simulink model "no_connections_stacey"  (R2023b)
settings: Solver=VariableStepAuto  StartTime=0.0  StopTime=20  RelTol=1e-3
undefined symbols (not defined in the file): delta_f, FF_gain, Fx200lbf, g, Izz, Kd, Ki, Kp, L, Lf, Lr, r_d_term, s, s_desired, T_down, T_request, T_switch, T_up, Tm_max, TV_switch, TV_vel_trig
libraries: slpidlib x2, Solver_SF x1, simulink x1, fuzblock x1
settings Model: Creator=savchenko.6  LastModifiedBy=savchenko.6
settings DataIOCC: ReturnWorkspaceOutputs=off
settings OptimizationCC: ReuseModelBlockBuffer=off

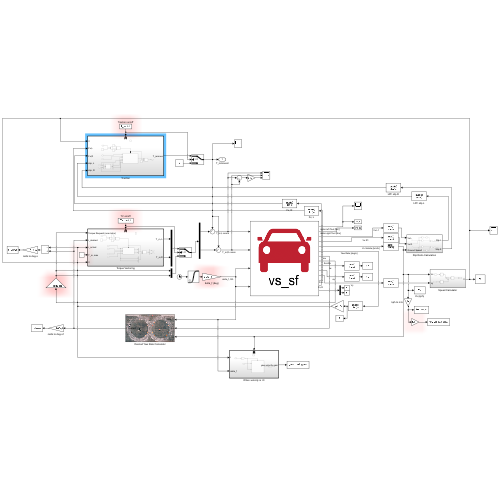
[thumbnail: Simulink's stored preview of the top-level diagram]
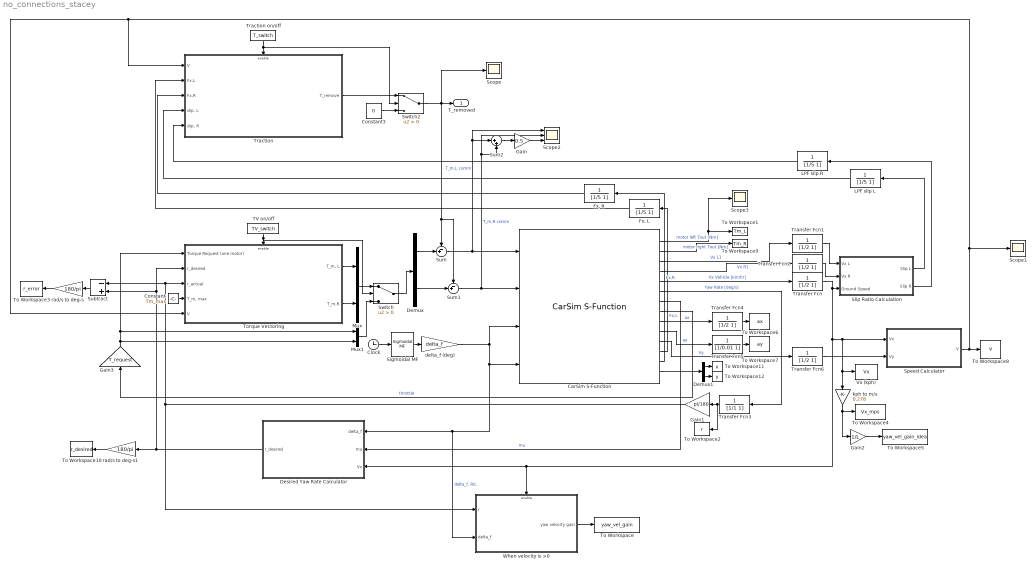
== system no_connections_stacey ==
  CarSim S-Function : Solver_SF/CarSim S-Function  Priority=1  SIMFILE=simfile.sim  Run_RTs=off  vs_state_ind=Run  StopMode_ind=Vehicle Model
  Clock : Clock
  Constant : Constant  Value=Tm_max
  Constant3 : Constant  Value=0
  Demux : Demux  Outputs=2
  Demux1 : Demux  Outputs=2
  Desired Yaw Rate Calculator : Subsystem
      mask Display: image('\\coeit.osu.edu\home\s\savchenko.6\Desktop\Capstone\Post-Depression\FB2018_Skidpad.png'); % Use "Edit Image" on toolstrip to change.
  "Fx, L" : TransferFcn  Denominator=[1/5 1]
  "Fx, R" : TransferFcn  Denominator=[1/5 1]
  Gain : Gain  Gain=0.5
  Gain1 : Gain  Gain=pi/180
  Gain2 : Gain  Gain=1/L
  Gain3 : Gain  Gain=T_request
  LPF slip L : TransferFcn  Denominator=[1/5 1]
  LPF slip R : TransferFcn  Denominator=[1/5 1]
  Mux : Mux  Inputs=2
  Mux1 : Mux  Inputs=2
  Scope : Scope
  Scope1 : Scope
  Scope2 : Scope  NumInputPorts=3
  Scope3 : Scope
  Sigmoidal MF : fuzblock/Membership  Functions/Sigmoidal MF  a=10  c=0.5
  Slip Ratio Calculation : Subsystem
  Speed Calculator : Subsystem
  Subtract : Sum  Inputs=-+
  Sum : Sum  Inputs=-+|
  Sum1 : Sum  Inputs=-+|
  Sum2 : Sum  Inputs=|++
  Switch : Switch  Criteria=u2 > Threshold  SaturateOnIntegerOverflow=off  InputSameDT=off
  Switch2 : Switch  Criteria=u2 > Threshold  SaturateOnIntegerOverflow=off  InputSameDT=off
  TV on/off : Constant  Value=TV_switch
  To Workspace : ToWorkspace  VariableName=yaw_vel_gain  SampleTime=-1
  To Workspace1 : ToWorkspace  VariableName=Tm_L  SampleTime=-1
  To Workspace10 : ToWorkspace  VariableName=r_desired  SampleTime=-1
  To Workspace11 : ToWorkspace  VariableName=x  SampleTime=-1
  To Workspace12 : ToWorkspace  VariableName=y  SampleTime=-1
  To Workspace2 : ToWorkspace  VariableName=r  SampleTime=-1
  To Workspace3 : ToWorkspace  VariableName=r_error  SampleTime=-1
  To Workspace4 : ToWorkspace  VariableName=Vx_mps  SampleTime=-1
  To Workspace5 : ToWorkspace  VariableName=yaw_vel_gain_ideal  SampleTime=-1
  To Workspace6 : ToWorkspace  VariableName=ax  SampleTime=-1
  To Workspace7 : ToWorkspace  VariableName=ay  SampleTime=-1
  To Workspace8 : ToWorkspace  VariableName=V  SampleTime=-1
  To Workspace9 : ToWorkspace  VariableName=Tm_R  SampleTime=-1
  Torque Vectoring : Subsystem  TreatAsAtomicUnit=on
  Traction : Subsystem  TreatAsAtomicUnit=on
  Traction on/off : Constant  Value=T_switch
  Transfer Fcn{,1..2,4,6} (5 alike) : TransferFcn  Denominator=[1/2 1]
  Transfer Fcn3 : TransferFcn  Denominator=[1/1 1]
  Transfer Fcn5 : TransferFcn  Denominator=[1/0.01 1]
  Vx (kph) : ToWorkspace  VariableName=Vx  SampleTime=-1
  When velocity is >0 : Subsystem  TreatAsAtomicUnit=on
  delta_f (deg) : Gain  Gain=delta_f
  kph to m/s : Gain  Gain=0.278
  rad/s to deg-s : Gain  Gain=180/pi
  rad/s to deg-s1 : Gain  Gain=180/pi
  T_removed : Outport
  wires:
  CarSim S-Function/5 -> Transfer Fcn/1  "Vx Vehicle [km/hr]"
  CarSim S-Function/6 -> Transfer Fcn3/1  "Yaw Rate [deg/s]"
  CarSim S-Function/7 -> Desired Yaw Rate Calculator/2(mu)  "mu"
  CarSim S-Function/3 -> Transfer Fcn1/1  "Vx L1"
  CarSim S-Function/4 -> Transfer Fcn2/1  "Vx R1"
  Slip Ratio Calculation/1(Slip L) -> LPF slip L/1
  Transfer Fcn/1 -> Speed Calculator/1(Vx), kph to m/s/1, Vx (kph)/1, Desired Yaw Rate Calculator/3(Vx), When velocity is >0/Enable, Slip Ratio Calculation/3(Ground Speed)
  Transfer Fcn1/1 -> Slip Ratio Calculation/1(Vx L)
  Transfer Fcn2/1 -> Slip Ratio Calculation/2(Vx R)
  TV on/off/1 -> Switch/2, Torque Vectoring/Enable
  Constant/1 -> Torque Vectoring/4("T_m, max")
  Torque Vectoring/2(T_m,R) -> Mux/2
  Torque Vectoring/1("T_m, L") -> Mux/1
  Mux/1 -> Switch/1
  Switch/1 -> Demux/1
  Mux1/1 -> Switch/3
  CarSim S-Function/8 -> Gain3/1  "throttle"
  When velocity is >0/1(yaw velocity gain) -> To Workspace/1
  Gain2/1 -> To Workspace5/1
  kph to m/s/1 -> Gain2/1, To Workspace4/1
  Subtract/1 -> rad/s to deg-s/1
  Gain3/1 -> Mux1/2, Mux1/1, Torque Vectoring/1(Torque Request (one motor))
  Traction/1(T_remove) -> Switch2/1
  Constant3/1 -> Switch2/3
  Traction on/off/1 -> Switch2/2, Traction/Enable
  Demux/2 -> Sum1/2
  Demux/1 -> Sum/2
  Switch2/1 -> Scope/1, Sum/1, Sum1/1, T_removed/1
  Sum1/1 -> Sum2/2, Scope2/2, CarSim S-Function/2  "T_m,R comm"
  Sum/1 -> Sum2/1, Scope2/1, CarSim S-Function/1  "T_m,L comm"
  CarSim S-Function/9 -> Transfer Fcn4/1  "ax"
  CarSim S-Function/10 -> Transfer Fcn5/1  "ay"
  Slip Ratio Calculation/2(Slip R) -> LPF slip R/1
  LPF slip L/1 -> Traction/4("slip, L")
  LPF slip R/1 -> Traction/5("slip, R")
  Gain1/1 -> When velocity is >0/1(r), Torque Vectoring/3(r_actual), Subtract/1
  Desired Yaw Rate Calculator/1(r_desired) -> rad/s to deg-s1/1, Torque Vectoring/2(r_desired), Subtract/2
  rad/s to deg-s/1 -> To Workspace3/1
  CarSim S-Function/11 -> Transfer Fcn6/1  "Vy"
  Transfer Fcn6/1 -> Speed Calculator/2(Vy)
  Speed Calculator/1(V) -> To Workspace8/1, Scope1/1, Torque Vectoring/5(V), Traction/1(V)
  CarSim S-Function/12 -> "Fx, L"/1  "Fx,L"
  CarSim S-Function/13 -> "Fx, R"/1  "Fx,R"
  Transfer Fcn4/1 -> To Workspace6/1
  Transfer Fcn5/1 -> To Workspace7/1
  CarSim S-Function/2 -> To Workspace9/1  "motor right Tout [Nm]"
  CarSim S-Function/1 -> Scope3/1, To Workspace1/1  "motor left Tout [Nm]"
  "Fx, R"/1 -> Traction/3(Fx,R)
  "Fx, L"/1 -> Traction/2(Fx,L)
  Transfer Fcn3/1 -> To Workspace2/1, Gain1/1
  rad/s to deg-s1/1 -> To Workspace10/1
  CarSim S-Function/14 -> Demux1/1
  Demux1/1 -> To Workspace11/1
  Demux1/2 -> To Workspace12/1
  delta_f (deg)/1 -> CarSim S-Function/3, When velocity is >0/2(delta_f), Desired Yaw Rate Calculator/1("delta_f "), CarSim S-Function/4  "delta_f, R/L"
  Sigmoidal MF/1 -> delta_f (deg)/1
  Clock/1 -> Sigmoidal MF/1
  Sum2/1 -> Gain/1
  Gain/1 -> Scope2/3

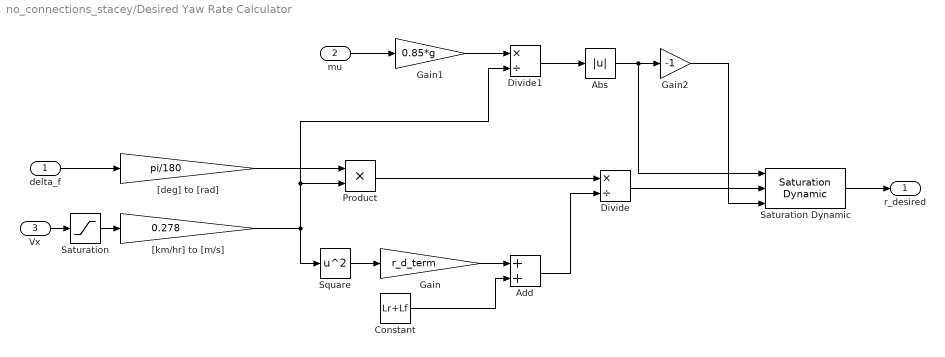
== system no_connections_stacey/Desired Yaw Rate Calculator ==
  "delta_f " : Inport
  mu : Inport  Port=2
  Vx : Inport  Port=3
  Abs : Abs  SaturateOnIntegerOverflow=off
  Add : Sum
  Constant : Constant  Value=Lr+Lf
  Divide : Product  Inputs=*/
  Divide1 : Product  Inputs=*/
  Gain : Gain  Gain=r_d_term
  Gain1 : Gain  Gain=0.85*g
  Gain2 : Gain  Gain=-1
  Product : Product
  Saturation : Saturate  UpperLimit=10000  LowerLimit=0.01
  Saturation Dynamic : simulink/Discontinuities/Saturation Dynamic  OutMin=[]  OutMax=[]  OutDataTypeStr=Inherit: Same as second input  OutDataType=fixdt(1, 16)  OutScaling=2^-10  DoSatur=off
  Square : Math  Operator=square
  "[deg] to [rad]" : Gain  Gain=pi/180
  "[km/hr] to [m/s]" : Gain  Gain=0.278
  r_desired : Outport
  wires:
  "delta_f "/1 -> "[deg] to [rad]"/1
  Vx/1 -> Saturation/1
  Saturation/1 -> "[km/hr] to [m/s]"/1
  "[deg] to [rad]"/1 -> Product/1
  "[km/hr] to [m/s]"/1 -> Square/1, Divide1/2, Product/2
  Product/1 -> Divide/1
  Square/1 -> Gain/1
  Gain/1 -> Add/1
  Constant/1 -> Add/2
  Add/1 -> Divide/2
  Divide/1 -> Saturation Dynamic/2
  Saturation Dynamic/1 -> r_desired/1
  mu/1 -> Gain1/1
  Gain1/1 -> Divide1/1
  Divide1/1 -> Abs/1
  Abs/1 -> Saturation Dynamic/1, Gain2/1
  Gain2/1 -> Saturation Dynamic/3

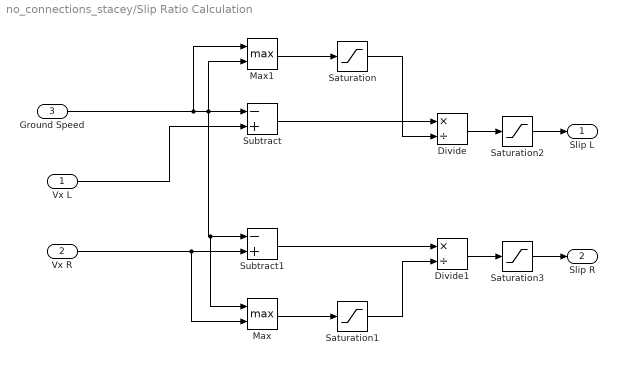
== system no_connections_stacey/Slip Ratio Calculation ==
  Vx L : Inport
  Vx R : Inport  Port=2
  Ground Speed : Inport  Port=3
  Divide : Product  Inputs=*/
  Divide1 : Product  Inputs=*/
  Max : MinMax  Function=max  Inputs=2
  Max1 : MinMax  Function=max  Inputs=2
  Saturation : Saturate  UpperLimit=1000  LowerLimit=0.0001
  Saturation1 : Saturate  UpperLimit=1000  LowerLimit=0.0001
  Saturation2 : Saturate  UpperLimit=1  LowerLimit=0
  Saturation3 : Saturate  UpperLimit=1  LowerLimit=0
  Subtract : Sum  Inputs=-+
  Subtract1 : Sum  Inputs=-+
  Slip L : Outport
  Slip R : Outport  Port=2
  wires:
  Vx L/1 -> Subtract/2
  Vx R/1 -> Max/2, Subtract1/2
  Max1/1 -> Saturation/1
  Max/1 -> Saturation1/1
  Subtract/1 -> Divide/1
  Saturation/1 -> Divide/2
  Subtract1/1 -> Divide1/1
  Saturation1/1 -> Divide1/2
  Divide/1 -> Saturation2/1
  Divide1/1 -> Saturation3/1
  Saturation2/1 -> Slip L/1
  Saturation3/1 -> Slip R/1
  Ground Speed/1 -> Max1/1, Max/1, Subtract1/1, Max1/2, Subtract/1

== system no_connections_stacey/Speed Calculator ==
  Vx : Inport
  Vy : Inport  Port=2
  Sqrt : Sqrt
  Square : Math  Operator=square
  Square1 : Math  Operator=square
  Sum : Sum  Inputs=|++
  V : Outport
  wires:
  Vx/1 -> Square/1
  Vy/1 -> Square1/1
  Square/1 -> Sum/1
  Square1/1 -> Sum/2
  Sum/1 -> Sqrt/1
  Sqrt/1 -> V/1

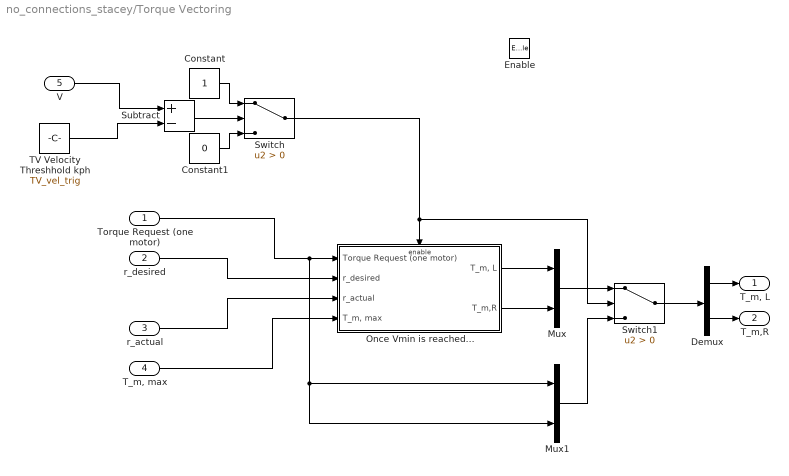
== system no_connections_stacey/Torque Vectoring ==
  Torque Request (one motor) : Inport
  r_desired : Inport  Port=2
  r_actual : Inport  Port=3
  "T_m, max" : Inport  Port=4
  V : Inport  Port=5
  Enable : EnablePort  StatesWhenEnabling=reset
  Constant : Constant
  Constant1 : Constant  Value=0
  Demux : Demux  Outputs=2
  Mux : Mux  Inputs=2
  Mux1 : Mux  Inputs=2
  Once Vmin is reached... : Subsystem
  Subtract : Sum  Inputs=+-
  Switch : Switch  Criteria=u2 > Threshold  SaturateOnIntegerOverflow=off  InputSameDT=off
  Switch1 : Switch  Criteria=u2 > Threshold  SaturateOnIntegerOverflow=off  InputSameDT=off
  TV Velocity Threshhold kph : Constant  Value=TV_vel_trig
  "T_m, L" : Outport
  T_m,R : Outport  Port=2
  wires:
  Torque Request (one motor)/1 -> Mux1/2, Mux1/1, Once Vmin is reached.../1(Torque Request (one motor))
  r_desired/1 -> Once Vmin is reached.../2(r_desired)
  r_actual/1 -> Once Vmin is reached.../3(r_actual)
  "T_m, max"/1 -> Once Vmin is reached.../4("T_m, max")
  Once Vmin is reached.../1("T_m, L") -> Mux/1
  Once Vmin is reached.../2(T_m,R) -> Mux/2
  Mux/1 -> Switch1/1
  Mux1/1 -> Switch1/3
  Switch1/1 -> Demux/1
  Demux/1 -> "T_m, L"/1
  Demux/2 -> T_m,R/1
  Constant1/1 -> Switch/3
  Switch/1 -> Switch1/2, Once Vmin is reached.../Enable
  Constant/1 -> Switch/1
  TV Velocity Threshhold kph/1 -> Subtract/2
  Subtract/1 -> Switch/2
  V/1 -> Subtract/1

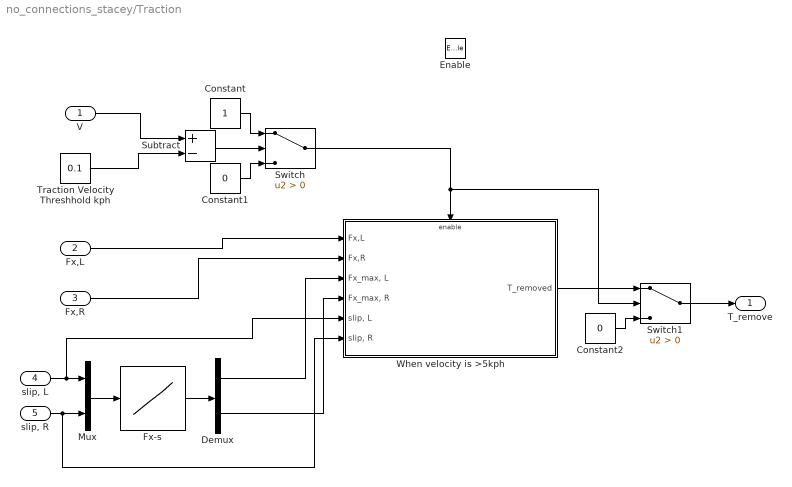
== system no_connections_stacey/Traction ==
  V : Inport
  Fx,L : Inport  Port=2
  Fx,R : Inport  Port=3
  "slip, L" : Inport  Port=4
  "slip, R" : Inport  Port=5
  Enable : EnablePort  StatesWhenEnabling=reset
  Constant : Constant
  Constant1 : Constant  Value=0
  Constant2 : Constant  Value=0
  Demux : Demux  Outputs=2
  Fx-s : Lookup_n-D  NumberOfTableDimensions=1  BreakpointsForDimension1=s  Table=Fx200lbf  InternalRulePriority=Speed  RndMeth=Simplest
  Mux : Mux  Inputs=2
  Subtract : Sum  Inputs=+-
  Switch : Switch  Criteria=u2 > Threshold  SaturateOnIntegerOverflow=off  InputSameDT=off
  Switch1 : Switch  Criteria=u2 > Threshold  SaturateOnIntegerOverflow=off  InputSameDT=off
  Traction Velocity Threshhold kph : Constant  Value=0.1
  When velocity is >5kph : Subsystem  TreatAsAtomicUnit=on
  T_remove : Outport
  wires:
  V/1 -> Subtract/1
  Traction Velocity Threshhold kph/1 -> Subtract/2
  Subtract/1 -> Switch/2
  Constant/1 -> Switch/1
  Constant1/1 -> Switch/3
  Switch/1 -> Switch1/2, When velocity is >5kph/Enable
  "slip, L"/1 -> When velocity is >5kph/5("slip, L"), Mux/1
  "slip, R"/1 -> When velocity is >5kph/6("slip, R"), Mux/2
  Mux/1 -> Fx-s/1
  Fx-s/1 -> Demux/1
  When velocity is >5kph/1(T_removed) -> Switch1/1
  Switch1/1 -> T_remove/1
  Constant2/1 -> Switch1/3
  Fx,L/1 -> When velocity is >5kph/1(Fx,L)
  Fx,R/1 -> When velocity is >5kph/2(Fx,R)
  Demux/1 -> When velocity is >5kph/3("Fx_max, L")
  Demux/2 -> When velocity is >5kph/4("Fx_max, R")

== system no_connections_stacey/When velocity is >0 ==
  r : Inport
  delta_f : Inport  Port=2
  Enable : EnablePort  StatesWhenEnabling=reset
  When Steering : Subsystem  TreatAsAtomicUnit=on
  deg to rad : Gain  Gain=pi/180
  yaw velocity gain : Outport
  wires:
  delta_f/1 -> deg to rad/1
  r/1 -> When Steering/1(r)
  When Steering/1(yaw velocity gain) -> yaw velocity gain/1
  deg to rad/1 -> When Steering/2(delta_f), When Steering/Enable

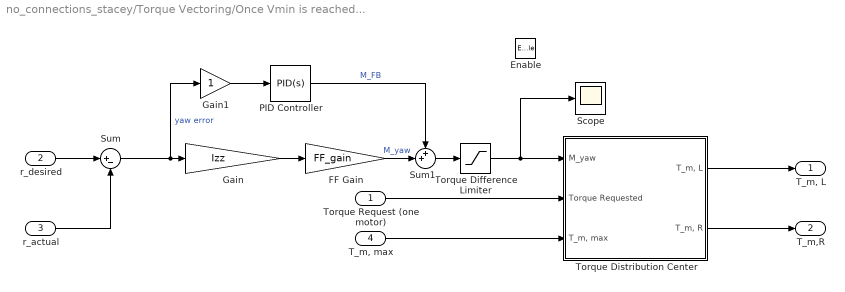
== system no_connections_stacey/Torque Vectoring/Once Vmin is reached... ==
  Torque Request (one motor) : Inport
  r_desired : Inport  Port=2
  r_actual : Inport  Port=3
  "T_m, max" : Inport  Port=4
  Enable : EnablePort  StatesWhenEnabling=reset
  FF Gain : Gain  Gain=FF_gain
  Gain : Gain  Gain=Izz
  Gain1 : Gain
  PID Controller : slpidlib/PID Controller  Controller=PID  Form=Parallel  TimeDomain=Continuous-time  UseExternalTs=off  SampleTime=-1  IntegratorMethod=Forward Euler  FilterMethod=Forward Euler  ControllerParametersSource=internal  P=Kp  I=Ki  UseKiTs=off  D=Kd  N=100  UseFilter=on  TunerSelectOption=Transfer Function Based (PID Tuner App)  InitialConditionSource=internal  InitialConditionForIntegrator=0  InitialConditionForFilter=0  DifferentiatorICPrevScaledInput=0  ExternalReset=none  TrackingMode=off  Kt=1  LimitOutput=off  SatLimitsSource=internal  UpperSaturationLimit=inf  LowerSaturationLimit=-inf  LinearizeAsGain=on  AntiWindupMode=none  Kb=1  LimitIntegrator=off  UpperIntegratorSaturationLimit=inf  LowerIntegratorSaturationLimit=-inf  POutMin=[]  POutMax=[]  IOutMin=[]  IOutMax=[]  DOutMin=[]  DOutMax=[]  NOutMin=[]  NOutMax=[]  SumOutMin=[]  SumOutMax=[]  SaturationOutMin=[]  SaturationOutMax=[]  PParamMin=[]  PParamMax=[]  IParamMin=[]  IParamMax=[]  DParamMin=[]  DParamMax=[]  NParamMin=[]  NParamMax=[]  KbParamMin=[]  KbParamMax=[]  KtParamMin=[]  KtParamMax=[]  KbOutMin=[]  KbOutMax=[]  KtOutMin=[]  KtOutMax=[]  IntegratorOutMin=[]  IntegratorOutMax=[]  FilterOutMin=[]  FilterOutMax=[]  SumI1OutMin=[]  SumI1OutMax=[]  SumI2OutMin=[]  SumI2OutMax=[]  SumI3OutMin=[]  SumI3OutMax=[]  SumI4OutMin=[]  SumI4OutMax=[]  SumDOutMin=[]  SumDOutMax=[]  DifferentiatorOutMin=[]  DifferentiatorOutMax=[]  FilterDiffOutCoefMin=[]  FilterDiffOutCoefMax=[]  ReciprocalOutMin=[]  ReciprocalOutMax=[]  SumDenOutMin=[]  SumDenOutMax=[]  SumNumOutMin=[]  SumNumOutMax=[]  DivideOutMin=[]  DivideOutMax=[]  UdiffTsProdOutMin=[]  UdiffTsProdOutMax=[]  NTsProdOutMin=[]  NTsProdOutMax=[]  UintegralTsProdOutMin=[]  UintegralTsProdOutMax=[]  UngainTsProdOutMin=[]  UngainTsProdOutMax=[]  ClampingZeroOutDataTypeStr=Inherit: Inherit via back propagation  ClampingZeroOutMin=[]  ClampingZeroOutMax=[]  FilterDenConstantOutDataTypeStr=Inherit: Inherit via back propagation  FilterDenConstantOutMin=[]  FilterDenConstantOutMax=[]  PCopyOutDataTypeStr=Inherit: Inherit via back propagation  PCopyOutMin=[]  PCopyOutMax=[]  NCopyOutDataTypeStr=Inherit: Inherit via back propagation  NCopyOutMin=[]  NCopyOutMax=[]  IntegratorContinuousStateAttributes=''  IntegratorStateMustResolveToSignalObject=off  IntegratorRTWStateStorageClass=Auto  FilterContinuousStateAttributes=''  FilterStateMustResolveToSignalObject=off  FilterRTWStateStorageClass=Auto  ParallelPVariant=InternalParameters  IdealPVariant=Disabled  IVariant=InternalParameters  DVariant=InternalParameters  IntegratorVariant=Continuous  SatVariant=Disabled  AWVariant=Passthrough  PCopyVariant=Disabled  TRVariant=Disabled  FdbkBlocksVariant=Forward  IdealPFdbkVariant=Disabled  SatFdbkVariant=Disabled  DerivativeFilterVariant=ContFilter  NVariant=InternalParameters  NCopyVariant=Disabled  FilterICVariant=InternalICsFilter  IntegratorICVariant=InternalICs  ExternalResetVariant=Disabled  TRSumVariant=Passthrough  SumFdbkVariant=Disabled  SumVariant=Sum_PID  TsampFilterVariant=InternalTs  TsampNgainVariant=Passthrough  TsampIntegralVariant=Disabled_SignalSpec  ExternalSaturationOutDataTypeStr=Inherit: Same as second input
  Scope : Scope
  Sum : Sum  Inputs=|+-
  Sum1 : Sum  Inputs=++|
  Torque Difference Limiter : Saturate  UpperLimit=T_up  LowerLimit=T_down
  Torque Distribution Center : Subsystem
  "T_m, L" : Outport
  T_m,R : Outport  Port=2
  wires:
  Torque Request (one motor)/1 -> Torque Distribution Center/2(Torque Requested)
  Gain/1 -> FF Gain/1
  Torque Difference Limiter/1 -> Scope/1, Torque Distribution Center/1(M_yaw)
  r_desired/1 -> Sum/1
  Torque Distribution Center/2("T_m, R") -> T_m,R/1
  Sum/1 -> Gain/1, Gain1/1  "yaw error"
  "T_m, max"/1 -> Torque Distribution Center/3("T_m, max")
  r_actual/1 -> Sum/2
  Torque Distribution Center/1("T_m, L") -> "T_m, L"/1
  Sum1/1 -> Torque Difference Limiter/1
  FF Gain/1 -> Sum1/2  "M_yaw"
  PID Controller/1 -> Sum1/1  "M_FB"
  Gain1/1 -> PID Controller/1

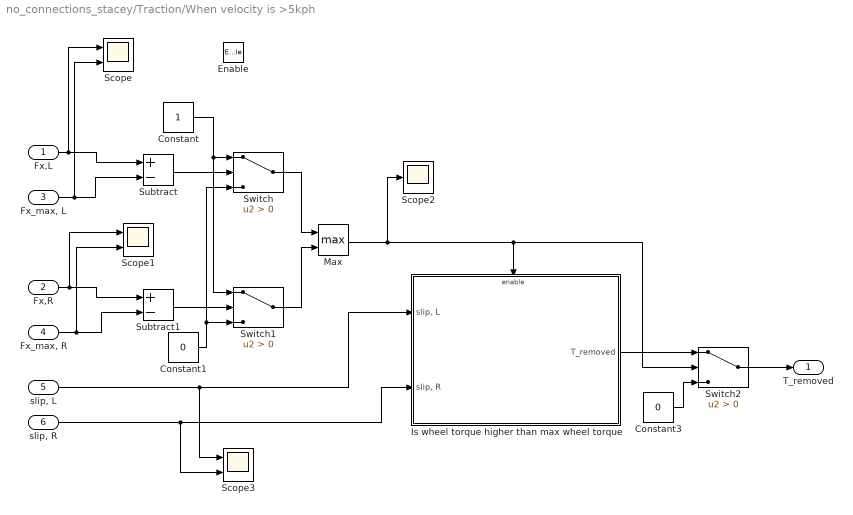
== system no_connections_stacey/Traction/When velocity is >5kph ==
  Fx,L : Inport
  Fx,R : Inport  Port=2
  "Fx_max, L" : Inport  Port=3
  "Fx_max, R" : Inport  Port=4
  "slip, L" : Inport  Port=5
  "slip, R" : Inport  Port=6
  Enable : EnablePort  StatesWhenEnabling=reset
  Constant : Constant
  Constant1 : Constant  Value=0
  Constant3 : Constant  Value=0
  Is wheel torque higher than max wheel torque : Subsystem  TreatAsAtomicUnit=on
  Max : MinMax  Function=max  Inputs=2
  Scope : Scope  NumInputPorts=2
  Scope1 : Scope  NumInputPorts=2
  Scope2 : Scope
  Scope3 : Scope  NumInputPorts=2
  Subtract : Sum  Inputs=+-
  Subtract1 : Sum  Inputs=+-
  Switch : Switch  Criteria=u2 > Threshold  SaturateOnIntegerOverflow=off  InputSameDT=off
  Switch1 : Switch  Criteria=u2 > Threshold  SaturateOnIntegerOverflow=off  InputSameDT=off
  Switch2 : Switch  Criteria=u2 > Threshold  SaturateOnIntegerOverflow=off  InputSameDT=off
  T_removed : Outport
  wires:
  Fx,L/1 -> Scope/1, Subtract/1
  "Fx_max, L"/1 -> Scope/2, Subtract/2
  "Fx_max, R"/1 -> Scope1/2, Subtract1/2
  Fx,R/1 -> Scope1/1, Subtract1/1
  Subtract/1 -> Switch/2
  Subtract1/1 -> Switch1/2
  Constant/1 -> Switch/1, Switch1/1
  Constant1/1 -> Switch1/3, Switch/3
  Switch/1 -> Max/1
  Switch1/1 -> Max/2
  Is wheel torque higher than max wheel torque/1(T_removed) -> Switch2/1
  Constant3/1 -> Switch2/3
  Max/1 -> Scope2/1, Is wheel torque higher than max wheel torque/Enable, Switch2/2
  Switch2/1 -> T_removed/1
  "slip, R"/1 -> Scope3/2, Is wheel torque higher than max wheel torque/2("slip, R")
  "slip, L"/1 -> Is wheel torque higher than max wheel torque/1("slip, L"), Scope3/1

== system no_connections_stacey/When velocity is >0/When Steering ==
  r : Inport
  delta_f : Inport  Port=2
  Enable : EnablePort  StatesWhenEnabling=reset
  Divide : Product  Inputs=*/
  yaw velocity gain : Outport
  wires:
  r/1 -> Divide/1
  delta_f/1 -> Divide/2
  Divide/1 -> yaw velocity gain/1

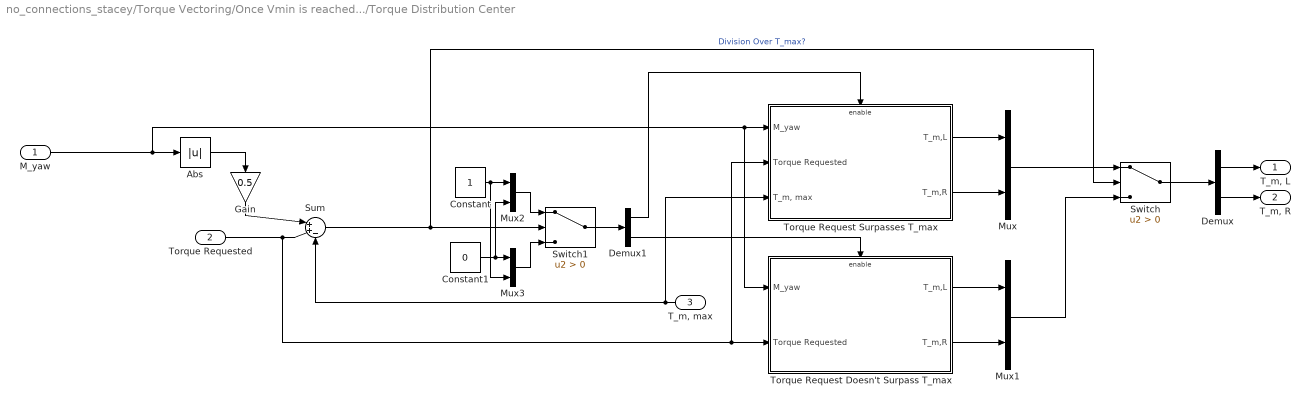
== system no_connections_stacey/Torque Vectoring/Once Vmin is reached.../Torque Distribution Center ==
  M_yaw : Inport
  Torque Requested : Inport  Port=2
  "T_m, max" : Inport  Port=3
  Abs : Abs  SaturateOnIntegerOverflow=off
  Constant : Constant
  Constant1 : Constant  Value=0
  Demux : Demux  Outputs=2
  Demux1 : Demux  Outputs=2
  Gain : Gain  Gain=0.5
  Mux{,1..3} (4 alike) : Mux  Inputs=2
  Sum : Sum  Inputs=|++-
  Switch : Switch  Criteria=u2 > Threshold  SaturateOnIntegerOverflow=off  InputSameDT=off
  Switch1 : Switch  Criteria=u2 > Threshold  SaturateOnIntegerOverflow=off  InputSameDT=off
  Torque Request Doesn't Surpass T_max : Subsystem  TreatAsAtomicUnit=on
  Torque Request Surpasses T_max : Subsystem  TreatAsAtomicUnit=on
  "T_m, L" : Outport
  "T_m, R" : Outport  Port=2
  wires:
  Sum/1 -> Switch1/2, Switch/2  "Division Over T_max?"
  Gain/1 -> Sum/1
  Abs/1 -> Gain/1
  Torque Request Surpasses T_max/1(T_m,L) -> Mux/1
  Torque Request Surpasses T_max/2(T_m,R) -> Mux/2
  Torque Request Doesn't Surpass T_max/1(T_m,L) -> Mux1/1
  Torque Request Doesn't Surpass T_max/2(T_m,R) -> Mux1/2
  Mux/1 -> Switch/1
  Mux1/1 -> Switch/3
  Switch/1 -> Demux/1
  Demux/1 -> "T_m, L"/1
  Demux/2 -> "T_m, R"/1
  Torque Requested/1 -> Torque Request Surpasses T_max/2(Torque Requested), Torque Request Doesn't Surpass T_max/2(Torque Requested), Sum/2
  "T_m, max"/1 -> Sum/3, Torque Request Surpasses T_max/3("T_m, max")
  Mux2/1 -> Switch1/1
  Mux3/1 -> Switch1/3
  Switch1/1 -> Demux1/1
  Demux1/1 -> Torque Request Surpasses T_max/Enable
  Demux1/2 -> Torque Request Doesn't Surpass T_max/Enable
  Constant/1 -> Mux2/1, Mux3/2
  Constant1/1 -> Mux2/2, Mux3/1
  M_yaw/1 -> Torque Request Doesn't Surpass T_max/1(M_yaw), Torque Request Surpasses T_max/1(M_yaw), Abs/1

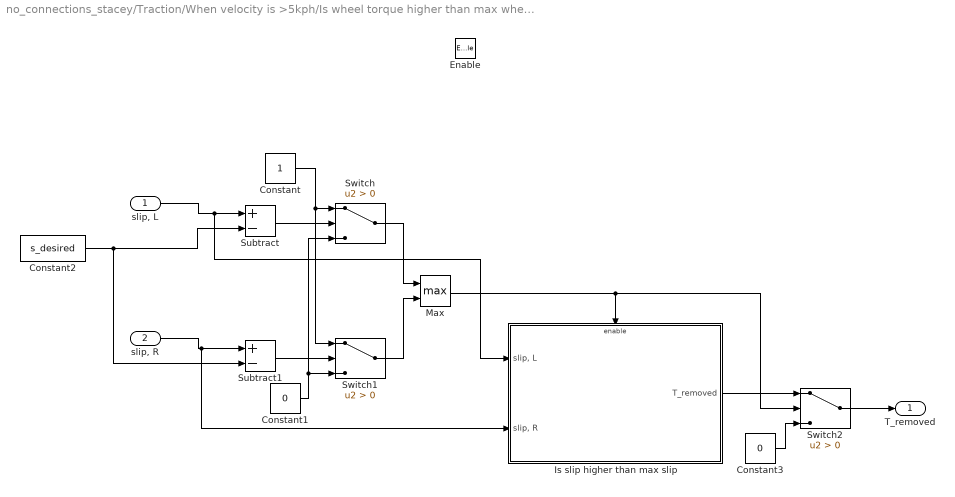
== system no_connections_stacey/Traction/When velocity is >5kph/Is wheel torque higher than max wheel torque ==
  "slip, L" : Inport
  "slip, R" : Inport  Port=2
  Enable : EnablePort  StatesWhenEnabling=reset
  Constant : Constant
  Constant1 : Constant  Value=0
  Constant2 : Constant  Value=s_desired
  Constant3 : Constant  Value=0
  Is slip higher than max slip : Subsystem  TreatAsAtomicUnit=on
  Max : MinMax  Function=max  Inputs=2
  Subtract : Sum  Inputs=+-
  Subtract1 : Sum  Inputs=+-
  Switch : Switch  Criteria=u2 > Threshold  SaturateOnIntegerOverflow=off  InputSameDT=off
  Switch1 : Switch  Criteria=u2 > Threshold  SaturateOnIntegerOverflow=off  InputSameDT=off
  Switch2 : Switch  Criteria=u2 > Threshold  SaturateOnIntegerOverflow=off  InputSameDT=off
  T_removed : Outport
  wires:
  Constant1/1 -> Switch1/3, Switch/3
  Max/1 -> Is slip higher than max slip/Enable, Switch2/2
  Subtract/1 -> Switch/2
  Switch/1 -> Max/1
  Constant2/1 -> Subtract1/2, Subtract/2
  "slip, R"/1 -> Is slip higher than max slip/2("slip, R"), Subtract1/1
  Constant/1 -> Switch/1, Switch1/1
  "slip, L"/1 -> Is slip higher than max slip/1("slip, L"), Subtract/1
  Switch1/1 -> Max/2
  Subtract1/1 -> Switch1/2
  Is slip higher than max slip/1(T_removed) -> Switch2/1
  Constant3/1 -> Switch2/3
  Switch2/1 -> T_removed/1

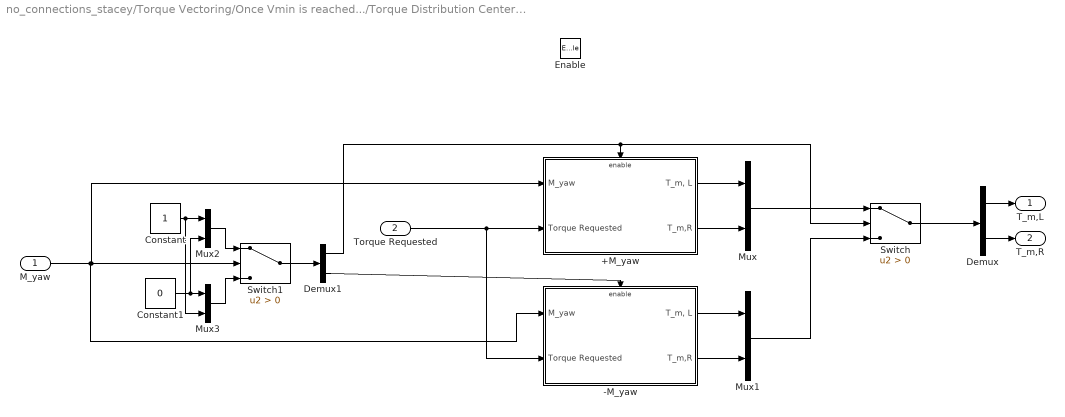
== system no_connections_stacey/Torque Vectoring/Once Vmin is reached.../Torque Distribution Center/Torque Request Doesn't Surpass T_max ==
  M_yaw : Inport
  Torque Requested : Inport  Port=2
  Enable : EnablePort  StatesWhenEnabling=reset
  +M_yaw : Subsystem  TreatAsAtomicUnit=on
  -M_yaw : Subsystem  TreatAsAtomicUnit=on
  Constant : Constant
  Constant1 : Constant  Value=0
  Demux : Demux  Outputs=2
  Demux1 : Demux  Outputs=2
  Mux{,1..3} (4 alike) : Mux  Inputs=2
  Switch : Switch  Criteria=u2 > Threshold  SaturateOnIntegerOverflow=off  InputSameDT=off
  Switch1 : Switch  Criteria=u2 > Threshold  SaturateOnIntegerOverflow=off  InputSameDT=off
  T_m,L : Outport
  T_m,R : Outport  Port=2
  wires:
  +M_yaw/1("T_m, L") -> Mux/1
  +M_yaw/2(T_m,R) -> Mux/2
  -M_yaw/1("T_m, L") -> Mux1/1
  -M_yaw/2(T_m,R) -> Mux1/2
  Mux/1 -> Switch/1
  Mux1/1 -> Switch/3
  Torque Requested/1 -> -M_yaw/2(Torque Requested), +M_yaw/2(Torque Requested)
  Switch/1 -> Demux/1
  Demux/1 -> T_m,L/1
  Demux/2 -> T_m,R/1
  Mux2/1 -> Switch1/1
  Demux1/1 -> Switch/2, +M_yaw/Enable
  Demux1/2 -> -M_yaw/Enable
  Mux3/1 -> Switch1/3
  Switch1/1 -> Demux1/1
  Constant1/1 -> Mux2/2, Mux3/1
  Constant/1 -> Mux2/1, Mux3/2
  M_yaw/1 -> Switch1/2, +M_yaw/1(M_yaw), -M_yaw/1(M_yaw)

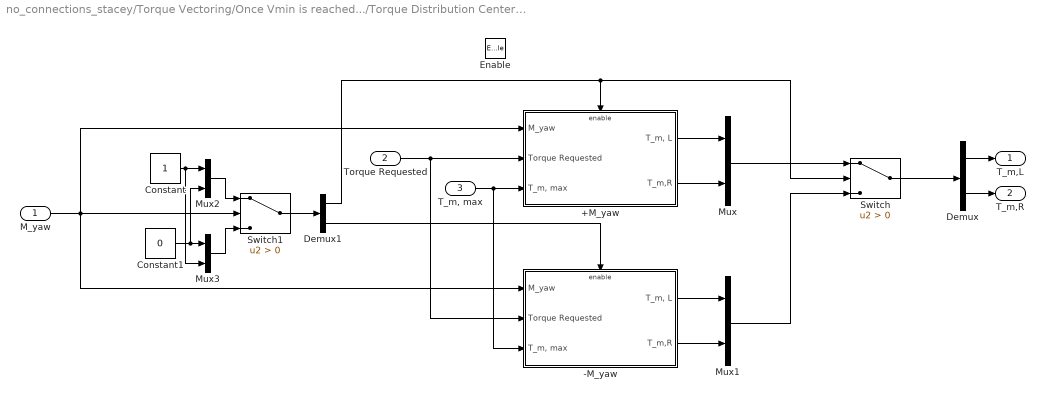
== system no_connections_stacey/Torque Vectoring/Once Vmin is reached.../Torque Distribution Center/Torque Request Surpasses T_max ==
  M_yaw : Inport
  Torque Requested : Inport  Port=2
  "T_m, max" : Inport  Port=3
  Enable : EnablePort  StatesWhenEnabling=reset
  +M_yaw : Subsystem  TreatAsAtomicUnit=on
  -M_yaw : Subsystem  TreatAsAtomicUnit=on
  Constant : Constant
  Constant1 : Constant  Value=0
  Demux : Demux  Outputs=2
  Demux1 : Demux  Outputs=2
  Mux{,1..3} (4 alike) : Mux  Inputs=2
  Switch : Switch  Criteria=u2 > Threshold  SaturateOnIntegerOverflow=off  InputSameDT=off
  Switch1 : Switch  Criteria=u2 > Threshold  SaturateOnIntegerOverflow=off  InputSameDT=off
  T_m,L : Outport
  T_m,R : Outport  Port=2
  wires:
  Mux/1 -> Switch/1
  Mux1/1 -> Switch/3
  Torque Requested/1 -> -M_yaw/2(Torque Requested), +M_yaw/2(Torque Requested)
  Demux/2 -> T_m,R/1
  Demux/1 -> T_m,L/1
  +M_yaw/2(T_m,R) -> Mux/2
  +M_yaw/1("T_m, L") -> Mux/1
  -M_yaw/2(T_m,R) -> Mux1/2
  Switch/1 -> Demux/1
  "T_m, max"/1 -> -M_yaw/3("T_m, max"), +M_yaw/3("T_m, max")
  -M_yaw/1("T_m, L") -> Mux1/1
  Mux2/1 -> Switch1/1
  Demux1/1 -> +M_yaw/Enable, Switch/2
  Demux1/2 -> -M_yaw/Enable
  Mux3/1 -> Switch1/3
  Switch1/1 -> Demux1/1
  Constant1/1 -> Mux2/2, Mux3/1
  Constant/1 -> Mux2/1, Mux3/2
  M_yaw/1 -> Switch1/2, -M_yaw/1(M_yaw), +M_yaw/1(M_yaw)

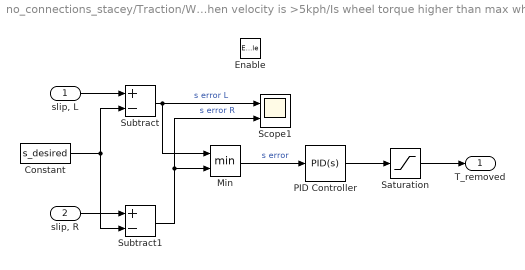
== system no_connections_stacey/Traction/When velocity is >5kph/Is wheel torque higher than max wheel torque/Is slip higher than max slip ==
  "slip, L" : Inport
  "slip, R" : Inport  Port=2
  Enable : EnablePort  StatesWhenEnabling=reset
  Constant : Constant  Value=s_desired
  Min : MinMax  Inputs=2
  PID Controller : slpidlib/PID Controller  Controller=PID  Form=Parallel  TimeDomain=Continuous-time  UseExternalTs=off  SampleTime=-1  IntegratorMethod=Forward Euler  FilterMethod=Forward Euler  ControllerParametersSource=internal  P=2  I=1  UseKiTs=off  D=0  N=100  UseFilter=on  TunerSelectOption=Transfer Function Based (PID Tuner App)  InitialConditionSource=internal  InitialConditionForIntegrator=0  InitialConditionForFilter=0  DifferentiatorICPrevScaledInput=0  ExternalReset=none  TrackingMode=off  Kt=1  LimitOutput=off  SatLimitsSource=internal  UpperSaturationLimit=inf  LowerSaturationLimit=-inf  LinearizeAsGain=on  AntiWindupMode=none  Kb=1  LimitIntegrator=off  UpperIntegratorSaturationLimit=inf  LowerIntegratorSaturationLimit=-inf  POutMin=[]  POutMax=[]  IOutMin=[]  IOutMax=[]  DOutMin=[]  DOutMax=[]  NOutMin=[]  NOutMax=[]  SumOutMin=[]  SumOutMax=[]  SaturationOutMin=[]  SaturationOutMax=[]  PParamMin=[]  PParamMax=[]  IParamMin=[]  IParamMax=[]  DParamMin=[]  DParamMax=[]  NParamMin=[]  NParamMax=[]  KbParamMin=[]  KbParamMax=[]  KtParamMin=[]  KtParamMax=[]  KbOutMin=[]  KbOutMax=[]  KtOutMin=[]  KtOutMax=[]  IntegratorOutMin=[]  IntegratorOutMax=[]  FilterOutMin=[]  FilterOutMax=[]  SumI1OutMin=[]  SumI1OutMax=[]  SumI2OutMin=[]  SumI2OutMax=[]  SumI3OutMin=[]  SumI3OutMax=[]  SumI4OutMin=[]  SumI4OutMax=[]  SumDOutMin=[]  SumDOutMax=[]  DifferentiatorOutMin=[]  DifferentiatorOutMax=[]  FilterDiffOutCoefMin=[]  FilterDiffOutCoefMax=[]  ReciprocalOutMin=[]  ReciprocalOutMax=[]  SumDenOutMin=[]  SumDenOutMax=[]  SumNumOutMin=[]  SumNumOutMax=[]  DivideOutMin=[]  DivideOutMax=[]  UdiffTsProdOutMin=[]  UdiffTsProdOutMax=[]  NTsProdOutMin=[]  NTsProdOutMax=[]  UintegralTsProdOutMin=[]  UintegralTsProdOutMax=[]  UngainTsProdOutMin=[]  UngainTsProdOutMax=[]  ClampingZeroOutDataTypeStr=Inherit: Inherit via back propagation  ClampingZeroOutMin=[]  ClampingZeroOutMax=[]  FilterDenConstantOutDataTypeStr=Inherit: Inherit via back propagation  FilterDenConstantOutMin=[]  FilterDenConstantOutMax=[]  PCopyOutDataTypeStr=Inherit: Inherit via back propagation  PCopyOutMin=[]  PCopyOutMax=[]  NCopyOutDataTypeStr=Inherit: Inherit via back propagation  NCopyOutMin=[]  NCopyOutMax=[]  IntegratorContinuousStateAttributes=''  IntegratorStateMustResolveToSignalObject=off  IntegratorRTWStateStorageClass=Auto  FilterContinuousStateAttributes=''  FilterStateMustResolveToSignalObject=off  FilterRTWStateStorageClass=Auto  ParallelPVariant=InternalParameters  IdealPVariant=Disabled  IVariant=InternalParameters  DVariant=InternalParameters  IntegratorVariant=Continuous  SatVariant=Disabled  AWVariant=Passthrough  PCopyVariant=Disabled  TRVariant=Disabled  FdbkBlocksVariant=Forward  IdealPFdbkVariant=Disabled  SatFdbkVariant=Disabled  DerivativeFilterVariant=ContFilter  NVariant=InternalParameters  NCopyVariant=Disabled  FilterICVariant=InternalICsFilter  IntegratorICVariant=InternalICs  ExternalResetVariant=Disabled  TRSumVariant=Passthrough  SumFdbkVariant=Disabled  SumVariant=Sum_PID  TsampFilterVariant=InternalTs  TsampNgainVariant=Passthrough  TsampIntegralVariant=Disabled_SignalSpec  ExternalSaturationOutDataTypeStr=Inherit: Same as second input
  Saturation : Saturate  UpperLimit=5  LowerLimit=0
  Scope1 : Scope  NumInputPorts=2
  Subtract : Sum  Inputs=+-
  Subtract1 : Sum  Inputs=+-
  T_removed : Outport
  wires:
  "slip, L"/1 -> Subtract/1
  "slip, R"/1 -> Subtract1/1
  Constant/1 -> Subtract/2, Subtract1/2
  Subtract/1 -> Scope1/1, Min/1  "s error L"
  Subtract1/1 -> Min/2, Scope1/2  "s error R"
  Min/1 -> PID Controller/1  "s error"
  PID Controller/1 -> Saturation/1
  Saturation/1 -> T_removed/1

== system no_connections_stacey/Torque Vectoring/Once Vmin is reached.../Torque Distribution Center/Torque Request Doesn't Surpass T_max/+M_yaw ==
  M_yaw : Inport
  Torque Requested : Inport  Port=2
  Enable : EnablePort  StatesWhenEnabling=reset
  Abs : Abs  SaturateOnIntegerOverflow=off
  Add : Sum
  Gain : Gain  Gain=0.5
  Subtract : Sum  Inputs=+-
  "T_m, L" : Outport
  T_m,R : Outport  Port=2
  wires:
  M_yaw/1 -> Abs/1
  Abs/1 -> Gain/1
  Gain/1 -> Add/2, Subtract/2
  Torque Requested/1 -> Subtract/1, Add/1
  Subtract/1 -> "T_m, L"/1
  Add/1 -> T_m,R/1

== system no_connections_stacey/Torque Vectoring/Once Vmin is reached.../Torque Distribution Center/Torque Request Doesn't Surpass T_max/-M_yaw ==
  M_yaw : Inport
  Torque Requested : Inport  Port=2
  Enable : EnablePort  StatesWhenEnabling=reset
  Abs : Abs  SaturateOnIntegerOverflow=off
  Add : Sum
  Gain : Gain  Gain=0.5
  Subtract : Sum  Inputs=+-
  "T_m, L" : Outport
  T_m,R : Outport  Port=2
  wires:
  Torque Requested/1 -> Subtract/1, Add/1
  Abs/1 -> Gain/1
  Gain/1 -> Add/2, Subtract/2
  M_yaw/1 -> Abs/1
  Subtract/1 -> T_m,R/1
  Add/1 -> "T_m, L"/1

== system no_connections_stacey/Torque Vectoring/Once Vmin is reached.../Torque Distribution Center/Torque Request Surpasses T_max/+M_yaw ==
  M_yaw : Inport
  Torque Requested : Inport  Port=2
  "T_m, max" : Inport  Port=3
  Enable : EnablePort  StatesWhenEnabling=reset
  Abs : Abs  SaturateOnIntegerOverflow=off
  Subtract : Sum  Inputs=+-
  Subtract1 : Sum  Inputs=+-
  Subtract2 : Sum  Inputs=-+
  "T_m, L" : Outport
  T_m,R : Outport  Port=2
  wires:
  "T_m, max"/1 -> T_m,R/1, Subtract/1
  M_yaw/1 -> Abs/1
  Abs/1 -> Subtract1/1
  Torque Requested/1 -> Subtract2/2, Subtract/2
  Subtract/1 -> Subtract1/2
  Subtract1/1 -> Subtract2/1
  Subtract2/1 -> "T_m, L"/1

== system no_connections_stacey/Torque Vectoring/Once Vmin is reached.../Torque Distribution Center/Torque Request Surpasses T_max/-M_yaw ==
  M_yaw : Inport
  Torque Requested : Inport  Port=2
  "T_m, max" : Inport  Port=3
  Enable : EnablePort  StatesWhenEnabling=reset
  Abs : Abs  SaturateOnIntegerOverflow=off
  Subtract : Sum  Inputs=+-
  Subtract1 : Sum  Inputs=+-
  Subtract2 : Sum  Inputs=-+
  "T_m, L" : Outport
  T_m,R : Outport  Port=2
  wires:
  Torque Requested/1 -> Subtract2/2, Subtract/2
  "T_m, max"/1 -> "T_m, L"/1, Subtract/1
  Subtract/1 -> Subtract1/2
  M_yaw/1 -> Abs/1
  Subtract1/1 -> Subtract2/1
  Abs/1 -> Subtract1/1
  Subtract2/1 -> T_m,R/1
